simulink model "tanks"  (R2021b)
settings: Solver=VariableStepAuto  StartTime=0.0  StopTime=200  RelTol=1e-3
values from neighbouring files (symbols this model uses):
  F = tf([K_pid*(Ti+Td*Ti*N), K_pid*(Ti*N +1),K_pid*N],[Ti, Ti*N 0])    [control_design.m]
  uss = alpha2/beta*sqrt(2*g*tank_init_h2)*100/15    [control_design.m]
  yss = 40    [control_design.m]
undefined symbols (not defined in the file or in its folder): tank_A1, tank_a1, tank_A2, tank_a2, tank_H1, tank_H2, tank_init_h1, tank_init_h2, tank_Kpump
settings Model: LastModifiedBy=rivaa
settings OptimizationCC: BlockReduction=off  BooleanDataType=off
settings DebuggingCC: SaveWithParameterizedLinksMsg=none  UnderspecifiedInitializationDetection=Classic  MergeDetectMultiDrivingBlocksExec=none  SignalResolutionControl=TryResolveAllWithWarning
settings HardwareCC: TargetUnknown=on
settings ModelReferenceCC: PropagateSignalLabelsOutOfModel=off

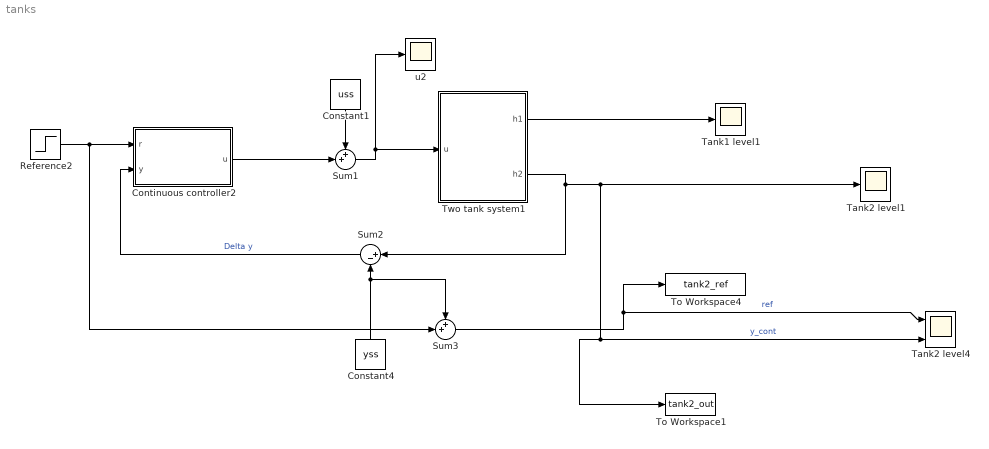
== system tanks ==
  Constant1 : Constant  Value=uss
  Constant4 : Constant  Value=yss
  Continuous controller2 : Subsystem
  Reference2 : Step  Time=25  After=10  SampleTime=0
  Sum1 : Sum  Inputs=++|
  Sum2 : Sum  Inputs=|+-
  Sum3 : Sum  Inputs=++|
  Tank1 level1 : Scope
  Tank2 level1 : Scope
  Tank2 level4 : Scope  NumInputPorts=2
  To Workspace1 : ToWorkspace  VariableName=tank2_out  SaveFormat=Structure With Time  SampleTime=-1
      settings: Save2DSignal=2-D array (concatenate along first dimension)
  To Workspace4 : ToWorkspace  VariableName=tank2_ref  SaveFormat=Timeseries  SampleTime=-1
      settings: Save2DSignal=2-D array (concatenate along first dimension)
  Two tank system1 : Subsystem
  u2 : Scope
  wires:
  Two tank system1/1(h1) -> Tank1 level1/1
  Constant1/1 -> Sum1/1
  Two tank system1/2(h2) -> Sum2/1, To Workspace1/1, Tank2 level4/2, Tank2 level1/1  "y_cont"
  Sum1/1 -> Two tank system1/1(u), u2/1
  Constant4/1 -> Sum3/1, Sum2/2
  Sum2/1 -> Continuous controller2/2(y)  "Delta y"
  Sum3/1 -> To Workspace4/1, Tank2 level4/1  "ref"
  Reference2/1 -> Continuous controller2/1(r), Sum3/2
  Continuous controller2/1(u) -> Sum1/2

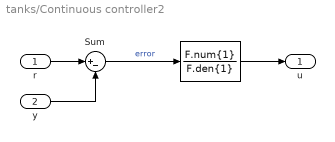
== system tanks/Continuous controller2 ==
  r : Inport
  y : Inport  Port=2
  " " : TransferFcn  Numerator=F.num{1}  Denominator=F.den{1}
  Sum : Sum  Inputs=|+-  SaturateOnIntegerOverflow=on
  u : Outport
  wires:
  Sum/1 -> " "/1  "error"
  y/1 -> Sum/2
  r/1 -> Sum/1
  " "/1 -> u/1

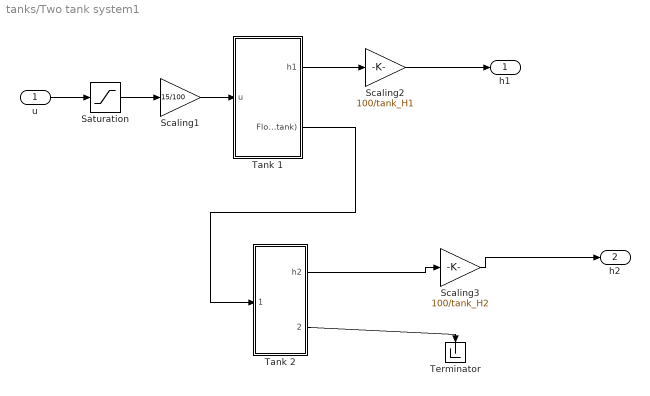
== system tanks/Two tank system1 ==
  u : Inport
  Saturation : Saturate  UpperLimit=100  LowerLimit=-0
  Scaling1 : Gain  Gain=15/100  SaturateOnIntegerOverflow=on  OutDataTypeStr=Inherit: Same as input  ParamDataTypeStr=Inherit: Same as input
  Scaling2 : Gain  Gain=100/tank_H1  SaturateOnIntegerOverflow=on  OutDataTypeStr=Inherit: Same as input  ParamDataTypeStr=Inherit: Same as input
  Scaling3 : Gain  Gain=100/tank_H2  SaturateOnIntegerOverflow=on  OutDataTypeStr=Inherit: Same as input  ParamDataTypeStr=Inherit: Same as input
  Tank 1 : Subsystem
  Tank 2 : Subsystem
  Terminator : Terminator
  h1 : Outport
  h2 : Outport  Port=2
  wires:
  Saturation/1 -> Scaling1/1
  Scaling1/1 -> Tank 1/1(u)
  Scaling3/1 -> h2/1
  Scaling2/1 -> h1/1
  Tank 1/2(Flow out  (to lower tank)) -> Tank 2/1(From upper tank)
  Tank 1/1(h1) -> Scaling2/1
  u/1 -> Saturation/1
  Tank 2/2(Flow out) -> Terminator/1
  Tank 2/1(h2) -> Scaling3/1

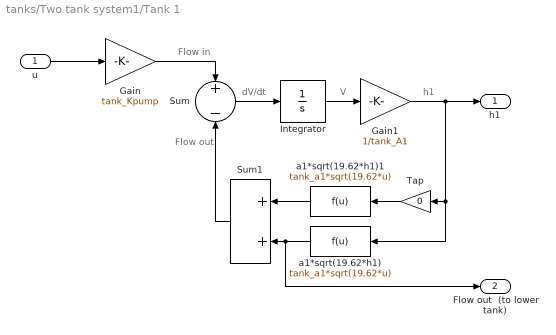
== system tanks/Two tank system1/Tank 1 ==
  note: Flow in
  note: Flow out
  note: dV/dt
  note: V
  note: h1
  u : Inport
  Gain : Gain  Gain=tank_Kpump  SaturateOnIntegerOverflow=on  OutDataTypeStr=Inherit: Same as input  ParamDataTypeStr=Inherit: Same as input
  Gain1 : Gain  Gain=1/tank_A1  SaturateOnIntegerOverflow=on  OutDataTypeStr=Inherit: Same as input  ParamDataTypeStr=Inherit: Same as input
  Integrator : Integrator  InitialCondition=tank_init_h1*tank_A1  LimitOutput=on  UpperSaturationLimit=tank_H1*tank_A1  LowerSaturationLimit=0
  Sum : Sum  Inputs=+-  InputSameDT=on  SaturateOnIntegerOverflow=on  OutDataTypeStr=Inherit: Same as first input
  Sum1 : Sum  InputSameDT=on  SaturateOnIntegerOverflow=on  OutDataTypeStr=Inherit: Same as first input
  Tap : Gain  Gain=0  SaturateOnIntegerOverflow=on  OutDataTypeStr=Inherit: Same as input  ParamDataTypeStr=Inherit: Same as input
  a1*sqrt(19.62*h1) : Fcn  Expr=tank_a1*sqrt(19.62*u)
  a1*sqrt(19.62*h1)1 : Fcn  Expr=tank_a1*sqrt(19.62*u)
  h1 : Outport
  Flow out  (to lower tank) : Outport  Port=2
  wires:
  Tap/1 -> a1*sqrt(19.62*h1)1/1
  Sum1/1 -> Sum/2
  a1*sqrt(19.62*h1)1/1 -> Sum1/1
  a1*sqrt(19.62*h1)/1 -> Sum1/2, Flow out  (to lower tank)/1
  u/1 -> Gain/1
  Gain/1 -> Sum/1
  Sum/1 -> Integrator/1
  Integrator/1 -> Gain1/1
  Gain1/1 -> h1/1, a1*sqrt(19.62*h1)/1, Tap/1

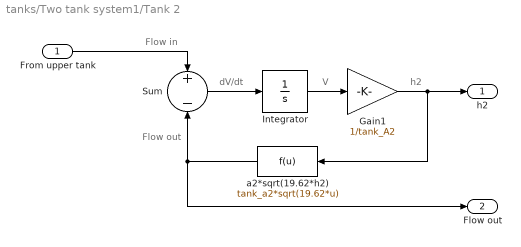
== system tanks/Two tank system1/Tank 2 ==
  note: h2
  note: V
  note: dV/dt
  note: Flow out
  note: Flow in
  From upper tank : Inport
  Gain1 : Gain  Gain=1/tank_A2  SaturateOnIntegerOverflow=on  OutDataTypeStr=Inherit: Same as input  ParamDataTypeStr=Inherit: Same as input
  Integrator : Integrator  InitialCondition=tank_init_h2*tank_A2  LimitOutput=on  UpperSaturationLimit=tank_H2*tank_A2  LowerSaturationLimit=0
  Sum : Sum  Inputs=+-  InputSameDT=on  SaturateOnIntegerOverflow=on  OutDataTypeStr=Inherit: Same as first input
  a2*sqrt(19.62*h2) : Fcn  Expr=tank_a2*sqrt(19.62*u)
  h2 : Outport
  Flow out : Outport  Port=2
  wires:
  From upper tank/1 -> Sum/1
  a2*sqrt(19.62*h2)/1 -> Flow out/1, Sum/2
  Gain1/1 -> a2*sqrt(19.62*h2)/1, h2/1
  Integrator/1 -> Gain1/1
  Sum/1 -> Integrator/1
